simulink model "model_2811_1"  (R2024b)
settings: Solver=VariableStepAuto  StartTime=0.0  StopTime=10.0  RelTol=1e-3
values from neighbouring files (symbols this model uses):
  f_v = 0.001    [Model_2811.m]
  Is = diag([0.06, 0.05, 0.06])    [satellite_Magtorq.m]
  Kd = 20    [Model_2811.m]    (also in sat_sim2711.m = diag([0.01, 0.01, 0.01]); satellitemodel2711.m = 1; untitled.m = 1)
  Ki = 0    [Model_2811.m]    (also in sat_sim2711.m = diag([0, 0, 0]); satellitemodel2711.m = 0.1; untitled.m = 10)
  Km = 0.01    [Model_2811.m]    (also in run_FIRST.m = 0.00574)
  Kp = 50    [Model_2811.m]    (also in sat_sim2711.m = diag([0.05, 0.05, 0.05]); satellitemodel2711.m = 10; untitled.m = 30)
  RWVmax = 3000 * (2*pi/60)    (= 314.159265359)    [Model_2811.m]
settings Model: Creator=LEGION  LastModifiedBy=LEGION

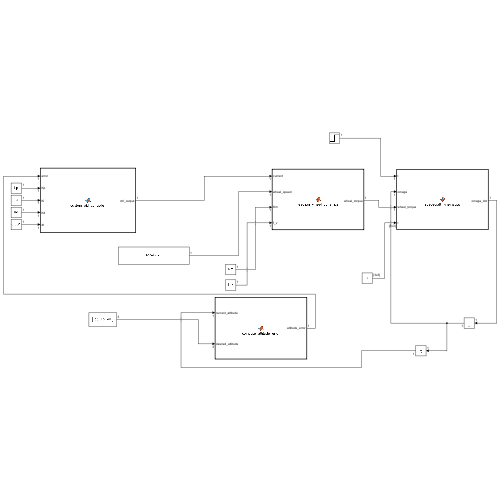
[thumbnail: Simulink's stored preview of the top-level diagram]
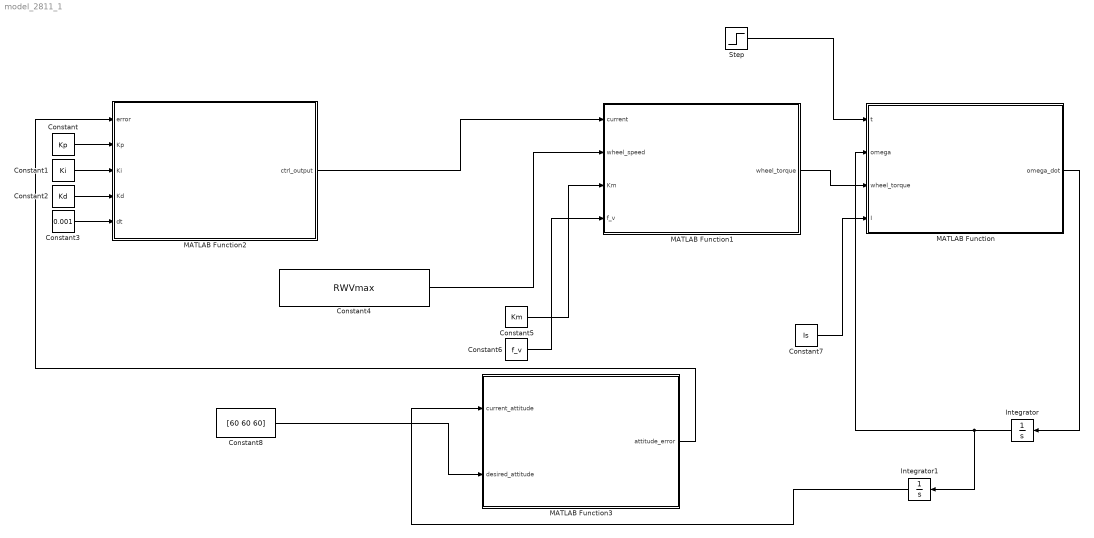
== system model_2811_1 ==
  Constant : Constant  Value=Kp
  Constant1 : Constant  Value=Ki
  Constant2 : Constant  Value=Kd
  Constant3 : Constant  Value=0.001
  Constant4 : Constant  Value=RWVmax
  Constant5 : Constant  Value=Km
  Constant6 : Constant  Value=f_v
  Constant7 : Constant  Value=Is
  Constant8 : Constant  Value=[60 60 60]
  Integrator : Integrator
  Integrator1 : Integrator
  MATLAB Function : MATLAB Function  TreatAsAtomicUnit=on
  MATLAB Function1 : MATLAB Function  TreatAsAtomicUnit=on
  MATLAB Function2 : MATLAB Function  TreatAsAtomicUnit=on
  MATLAB Function3 : MATLAB Function  TreatAsAtomicUnit=on
  Step : Step  SampleTime=0
  wires:
  Constant/1 -> MATLAB Function2/2(Kp)
  Constant1/1 -> MATLAB Function2/3(Ki)
  Constant2/1 -> MATLAB Function2/4(Kd)
  Constant3/1 -> MATLAB Function2/5(dt)
  MATLAB Function2/1(ctrl_output) -> MATLAB Function1/1(current)
  Constant4/1 -> MATLAB Function1/2(wheel_speed)
  Constant5/1 -> MATLAB Function1/3(Km)
  Constant6/1 -> MATLAB Function1/4(f_v)
  MATLAB Function1/1(wheel_torque) -> MATLAB Function/3(wheel_torque)
  Constant7/1 -> MATLAB Function/4(I)
  MATLAB Function/1(omega_dot) -> Integrator/1
  Integrator/1 -> Integrator1/1, MATLAB Function/2(omega)
  Step/1 -> MATLAB Function/1(t)
  MATLAB Function3/1(attitude_error) -> MATLAB Function2/1(error)
  Integrator1/1 -> MATLAB Function3/1(current_attitude)
  Constant8/1 -> MATLAB Function3/2(desired_attitude)

== matlab function model_2811_1/MATLAB Function1 ==
  data: current input; wheel_torque output; wheel_speed input; Km input; f_v input
%% 2. Reaction Wheel Dynamics Function
function wheel_torque  = reaction_wheel_dynamics(current, wheel_speed, Km, f_v)
    % Calculate reaction wheel torque based on input current
    % Inputs:
    %   current - input current to the wheel (A)
    %   wheel_speed - current wheel angular velocity (rad/s)
    %   params - struct containing wheel parameters
    
    % Calculate wheel torque
    % τ = Km * I - B * ω
    wheel_torque = Km * current - ...
                  f_v * wheel_speed;
    
    % Saturate torque to maximum wheel capability
    wheel_torque = max(-params.MaxTorque, min(params.MaxTorque, wheel_torque));
end

== matlab function model_2811_1/MATLAB Function ==
  data: t input; omega_dot output; omega input; wheel_torque input; I input
%% 1. Spacecraft Kinematics Function
function omega_dot  = spacecraft_kinematics(t, omega, wheel_torque, I)
    % Calculate spacecraft angular acceleration
    % Inputs:
    %   t - current time
    %   omega - current angular velocity vector [wx; wy; wz]
    %   wheel_torque - reaction wheel torque vector [Tx; Ty; Tz]
    %   I - moment of inertia matrix [Ix, 0, 0; 0, Iy, 0; 0, 0, Iz]
    
    % Define external disturbance torque (optional)
    % Simulates small random disturbances
    disturbance_torque = [0.01 * sin(t); 
                          0.02 * cos(t); 
                          0.005 * sin(2*t)];
    
    % Calculate angular acceleration using rigid body dynamics equation
    % ω̇ = I⁻¹ * (τ_wheel - ω × (I * ω) + τ_disturbance)
    omega_cross = [0, -omega(3), omega(2);
                   omega(3), 0, -omega(1);
                   -omega(2), omega(1), 0];
    
    % Compute angular acceleration
    omega_dot = inv(diag([I(1,1), I(2,2), I(3,3)])) * ...
        (wheel_torque - omega_cross * diag([I(1,1), I(2,2), I(3,3)]) * omega + disturbance_torque);
end

== matlab function model_2811_1/MATLAB Function2 ==
  data: error input; ctrl_output output; Kp input; Ki input; Kd input; dt input
%% 3. PID Controller Customization Function
function ctrl_output  = custom_pid_controller(error, Kp, Ki, Kd, dt)
    % Implements a custom PID controller with anti-windup
    % Inputs:
    %   error - control error
    %   Kp, Ki, Kd - PID gains
    %   dt - time step
    
    % Persistent variables to track integral and derivative terms
    persistent prev_error integral_term
    
    % Initialize persistent variables if not already set
    if isempty(prev_error)
        prev_error = 0;
        integral_term = 0;
    end
    
    % Proportional term
    P = Kp * error;
    
    % Integral term with anti-windup
    integral_term = integral_term + error * dt;
    I = Ki * integral_term;
    
    % Derivative term
    D = Kd * (error - prev_error) / dt;
    
    % Compute control output
    ctrl_output = P + I + D;
    
    % Update previous error
    prev_error = error;
end

== matlab function model_2811_1/MATLAB Function3 ==
  data: current_attitude input; attitude_error output; desired_attitude input
%% 4. Attitude Determination Function
function attitude_error  = compute_attitude_error(current_attitude, desired_attitude)
    % Compute attitude error between current and desired orientations
    % Uses quaternion representation or Euler angle difference
    
    % Simple error calculation (can be more complex depending on requirements)
    attitude_error = desired_attitude - current_attitude;
    
    % Normalize error to keep within reasonable bounds
    attitude_error = wrapToPi(attitude_error);
end
